simulink model "sub_1"  (Simulink 9.2)
settings: Solver=ode45  StartTime=0.0  StopTime=3  RelTol=1e-3  EnableMultiTasking=on
settings Model: Creator=student  LastModifiedBy=murad
settings OptimizationCC: ExpressionDepthLimit=2147483647
settings DebuggingCC: SolverPrmCheckMsg=warning

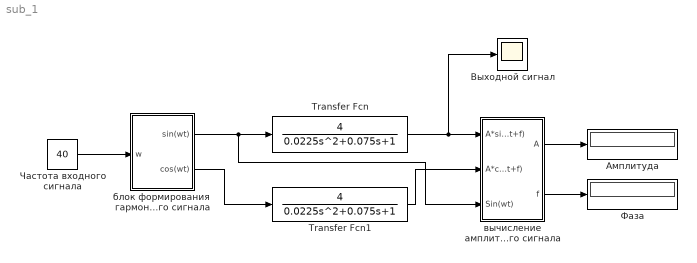
== system sub_1 ==
  Transfer Fcn : TransferFcn  Numerator=[4]  Denominator=[0.0225 0.075 1]
  Transfer Fcn1 : TransferFcn  Numerator=[4]  Denominator=[0.0225 0.075 1]
  Амплитуда : Display
  Выходной сигнал : Scope
  Фаза : Display
  Частота входного сигнала : Constant  Value=40
  блок формирования  гармонического сигнала : Subsystem
  "вычисление амплитуды и фазы выходного сигнала " : Subsystem
  wires:
  Частота входного сигнала/1 -> блок формирования  гармонического сигнала/1(w)
  блок формирования  гармонического сигнала/1(sin(wt)) -> Transfer Fcn/1, "вычисление амплитуды и фазы выходного сигнала "/3(Sin(wt))
  блок формирования  гармонического сигнала/2(cos(wt)) -> Transfer Fcn1/1
  Transfer Fcn/1 -> Выходной сигнал/1, "вычисление амплитуды и фазы выходного сигнала "/1(A*sin(wt+f))
  Transfer Fcn1/1 -> "вычисление амплитуды и фазы выходного сигнала "/2(A*cos(wt+f))
  "вычисление амплитуды и фазы выходного сигнала "/1(A) -> Амплитуда/1
  "вычисление амплитуды и фазы выходного сигнала "/2(f) -> Фаза/1

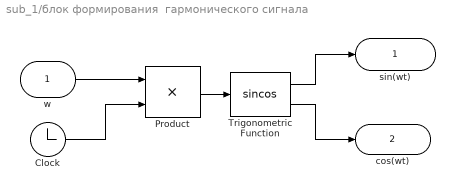
== system sub_1/блок формирования  гармонического сигнала ==
  w : Inport
  Clock : Clock
  Product : Product  RndMeth=Zero
  Trigonometric Function : Trigonometry  Operator=sincos
  sin(wt) : Outport
  cos(wt) : Outport  Port=2
  wires:
  Product/1 -> Trigonometric Function/1
  w/1 -> Product/1
  Clock/1 -> Product/2
  Trigonometric Function/1 -> sin(wt)/1
  Trigonometric Function/2 -> cos(wt)/1

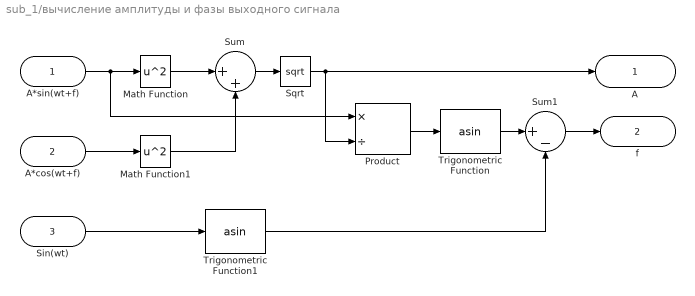
== system sub_1/вычисление амплитуды и фазы выходного сигнала  ==
  A*sin(wt+f) : Inport
  A*cos(wt+f) : Inport  Port=2
  Sin(wt) : Inport  Port=3
  Math Function : Math  Operator=square  SaturateOnIntegerOverflow=on
  Math Function1 : Math  Operator=square  SaturateOnIntegerOverflow=on
  Product : Product  Inputs=*/  RndMeth=Zero
  Sqrt : Sqrt  SaturateOnIntegerOverflow=on
  Sum : Sum  Inputs=|++
  Sum1 : Sum  Inputs=|+-
  Trigonometric Function : Trigonometry  Operator=asin
  Trigonometric Function1 : Trigonometry  Operator=asin
  A : Outport
  f : Outport  Port=2
  wires:
  A*sin(wt+f)/1 -> Math Function/1, Product/1
  Math Function/1 -> Sum/1
  Sum/1 -> Sqrt/1
  Sqrt/1 -> A/1, Product/2
  A*cos(wt+f)/1 -> Math Function1/1
  Math Function1/1 -> Sum/2
  Product/1 -> Trigonometric Function/1
  Sum1/1 -> f/1
  Trigonometric Function/1 -> Sum1/1
  Trigonometric Function1/1 -> Sum1/2
  Sin(wt)/1 -> Trigonometric Function1/1
